simulink model "test_ring"  (R2013a)
settings: Solver=ode45  StartTime=0.0  StopTime=inf  RelTol=1e-3
libraries: teste_lib x10
settings Model: Creator=michelr  LastModifiedBy=michelr
settings SolverCC: AlgebraicLoopSolver=LineSearch

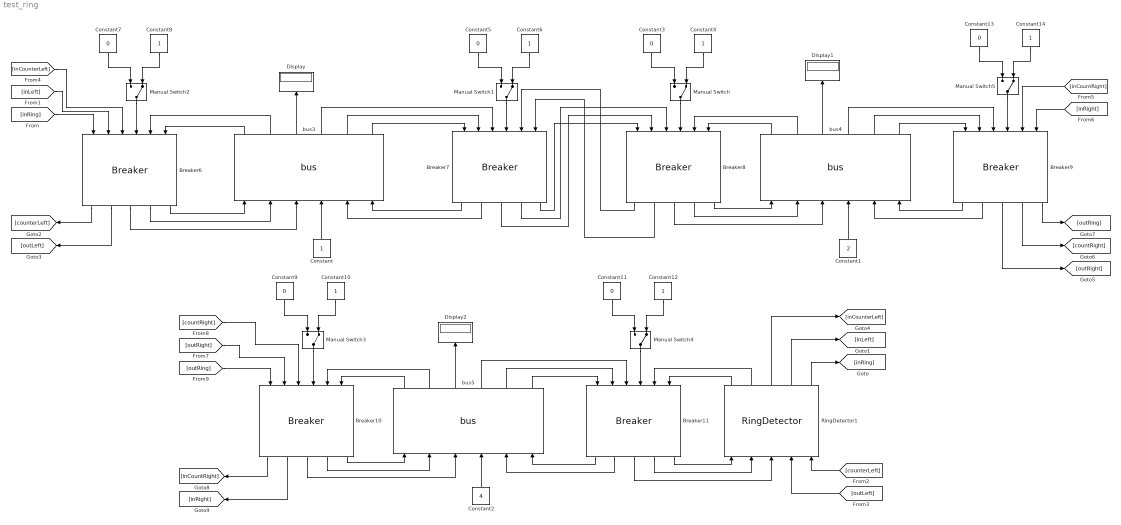
== system test_ring ==
  Breaker{6..11} (6 alike) : teste_lib/Breaker
  Constant{,4,6,8,10,12,14} (7 alike) : Constant
  Constant1 : Constant  Value=2
  Constant{3,5,7,9,11,13} (6 alike) : Constant  Value=0
  Constant2 : Constant  Value=4
  Display : Display
  Display1 : Display
  Display2 : Display
  Manual Switch{,1..5} (6 alike) : ManualSwitch  CurrentSetting=0
  RingDetector1 : teste_lib/RingDetector
  bus3 : teste_lib/bus
  bus4 : teste_lib/bus
  bus5 : teste_lib/bus
  wires:
  bus5/1 -> Breaker10/6
  bus5/2 -> Breaker10/5
  bus5/6 -> Breaker11/1
  bus5/5 -> Breaker11/2
  bus5/4 -> Breaker11/3
  Breaker11/1 -> bus5/6
  Breaker11/2 -> bus5/5
  Breaker11/5 -> RingDetector1/1
  Breaker11/4 -> RingDetector1/2
  Breaker11/3 -> RingDetector1/3
  RingDetector1/1 -> Breaker11/6
  RingDetector1/2 -> Breaker11/5
  Breaker10/5 -> bus5/1
  Breaker10/4 -> bus5/2
  Breaker10/3 -> bus5/3
  bus3/1 -> Breaker6/6
  bus3/2 -> Breaker6/5
  bus3/6 -> Breaker7/1
  bus3/5 -> Breaker7/2
  bus3/4 -> Breaker7/3
  Breaker6/5 -> bus3/1
  Breaker6/4 -> bus3/2
  Breaker6/3 -> bus3/3
  Breaker7/1 -> bus3/6
  Breaker7/2 -> bus3/5
  Breaker7/5 -> Breaker8/1
  Breaker7/4 -> Breaker8/3
  Breaker7/3 -> Breaker8/2
  Breaker8/2 -> Breaker7/6
  Breaker8/1 -> Breaker7/5
  bus4/1 -> Breaker8/6
  bus4/2 -> Breaker8/5
  Breaker8/5 -> bus4/1
  Breaker8/4 -> bus4/2
  Breaker8/3 -> bus4/3
  bus4/6 -> Breaker9/1
  bus4/5 -> Breaker9/2
  bus4/4 -> Breaker9/3
  Breaker9/1 -> bus4/6
  Breaker9/2 -> bus4/5
  bus3/3 -> Display/1
  bus4/3 -> Display1/1
  bus5/3 -> Display2/1
  Constant2/1 -> bus5/4
  Constant/1 -> bus3/4
  Constant1/1 -> bus4/4
  Constant3/1 -> Manual Switch/1
  Constant4/1 -> Manual Switch/2
  Manual Switch/1 -> Breaker8/4
  Constant5/1 -> Manual Switch1/1
  Constant6/1 -> Manual Switch1/2
  Manual Switch1/1 -> Breaker7/4
  Constant7/1 -> Manual Switch2/1
  Constant8/1 -> Manual Switch2/2
  Manual Switch2/1 -> Breaker6/4
  Constant9/1 -> Manual Switch3/1
  Constant10/1 -> Manual Switch3/2
  Manual Switch3/1 -> Breaker10/4
  Constant11/1 -> Manual Switch4/1
  Constant12/1 -> Manual Switch4/2
  Manual Switch4/1 -> Breaker11/4
  Breaker6/1 -> [counterLeft]
  Breaker6/2 -> [outLeft]
  [inRing] -> Breaker6/1
  [inLeft] -> Breaker6/2
  [inCounterLeft] -> Breaker6/3
  RingDetector1/5 -> [inRing]
  RingDetector1/4 -> [inLeft]
  RingDetector1/3 -> [inCounterLeft]
  [counterLeft] -> RingDetector1/5
  [outLeft] -> RingDetector1/4
  [inRight] -> Breaker9/6
  [inCountRight] -> Breaker9/5
  Breaker9/5 -> [outRing]
  Breaker9/4 -> [countRight]
  Breaker9/3 -> [outRight]
  [outRing] -> Breaker10/1
  [countRight] -> Breaker10/3
  [outRight] -> Breaker10/2
  Breaker10/1 -> [inCountRight]
  Breaker10/2 -> [inRight]
  Constant13/1 -> Manual Switch5/1
  Constant14/1 -> Manual Switch5/2
  Manual Switch5/1 -> Breaker9/4
